simulink model "q3"  (R2021b)
settings: Solver=VariableStepAuto  StartTime=0.0  StopTime=100  RelTol=1e-3
libraries: cstblocks x3
settings Model: Creator=Asus  LastModifiedBy=ASUS

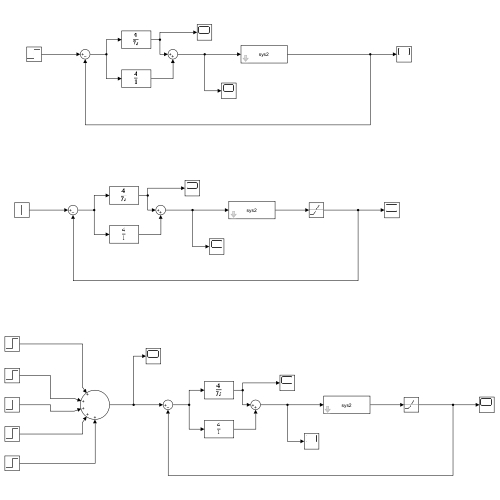
[thumbnail: Simulink's stored preview of the top-level diagram]
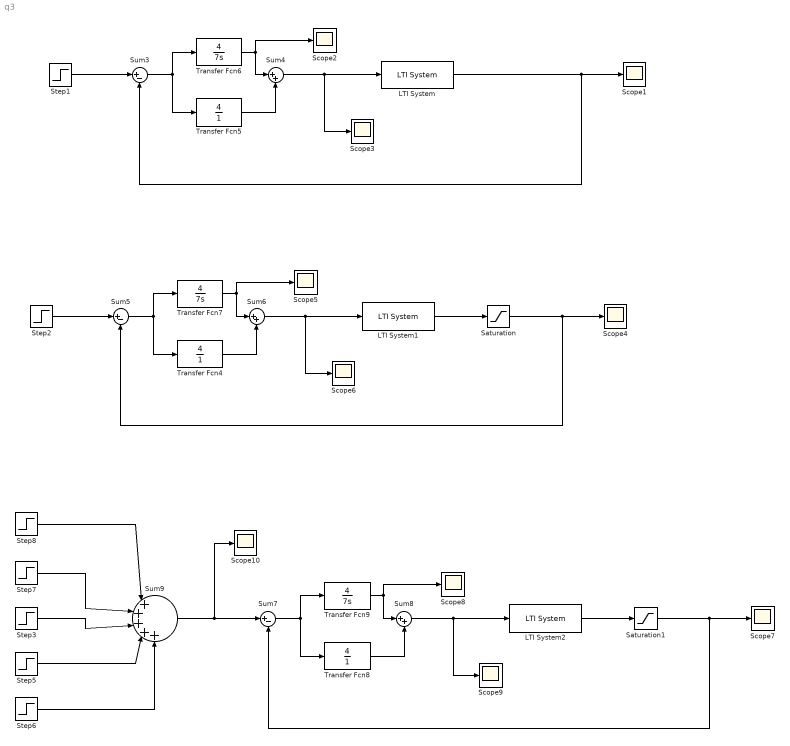
== system q3 ==
  LTI System : cstblocks/LTI System  sys=sys2  IC=[]
  LTI System1 : cstblocks/LTI System  sys=sys2  IC=[]
  LTI System2 : cstblocks/LTI System  sys=sys2  IC=[]
  Saturation : Saturate  UpperLimit=1.5  LowerLimit=-1.5
  Saturation1 : Saturate  UpperLimit=1.5  LowerLimit=-1.5
  Scope{1..10} (10 alike) : Scope
  Step1 : Step  SampleTime=0
  Step2 : Step  SampleTime=0
  Step3 : Step  Time=3  After=0.2  SampleTime=0
  Step5 : Step  Time=4  After=0.2  SampleTime=0
  Step6 : Step  Time=5  After=0.2  SampleTime=5
  Step7 : Step  Time=2  After=0.2  SampleTime=0
  Step8 : Step  After=0.2  SampleTime=0
  Sum3 : Sum  Inputs=|+-
  Sum4 : Sum  Inputs=|++
  Sum5 : Sum  Inputs=|+-
  Sum6 : Sum  Inputs=|++
  Sum7 : Sum  Inputs=|+-
  Sum8 : Sum  Inputs=|++
  Sum9 : Sum  Inputs=|+++++
  Transfer Fcn4 : TransferFcn  Numerator=[4]  Denominator=[1]
  Transfer Fcn5 : TransferFcn  Numerator=[4]  Denominator=[1]
  Transfer Fcn6 : TransferFcn  Numerator=[4]  Denominator=[7 0]
  Transfer Fcn7 : TransferFcn  Numerator=[4]  Denominator=[7 0]
  Transfer Fcn8 : TransferFcn  Numerator=[4]  Denominator=[1]
  Transfer Fcn9 : TransferFcn  Numerator=[4]  Denominator=[7 0]
  wires:
  Step3/1 -> Sum9/3
  Step5/1 -> Sum9/4
  Sum9/1 -> Scope10/1, Sum7/1
  Step6/1 -> Sum9/5
  Transfer Fcn7/1 -> Scope5/1, Sum6/1
  Sum8/1 -> LTI System2/1, Scope9/1
  Step7/1 -> Sum9/2
  Saturation1/1 -> Sum7/2, Scope7/1
  Step2/1 -> Sum5/1
  Sum3/1 -> Transfer Fcn5/1, Transfer Fcn6/1
  Sum6/1 -> LTI System1/1, Scope6/1
  Transfer Fcn6/1 -> Scope2/1, Sum4/1
  Sum4/1 -> LTI System/1, Scope3/1
  Saturation/1 -> Sum5/2, Scope4/1
  LTI System/1 -> Sum3/2, Scope1/1
  Transfer Fcn5/1 -> Sum4/2
  Step1/1 -> Sum3/1
  Step8/1 -> Sum9/1
  Transfer Fcn4/1 -> Sum6/2
  Sum5/1 -> Transfer Fcn4/1, Transfer Fcn7/1
  Sum7/1 -> Transfer Fcn8/1, Transfer Fcn9/1
  LTI System1/1 -> Saturation/1
  LTI System2/1 -> Saturation1/1
  Transfer Fcn9/1 -> Scope8/1, Sum8/1
  Transfer Fcn8/1 -> Sum8/2
